simulink model "MPPT2"  (R2018b)
settings: Solver=ode23tb  StartTime=0.0  StopTime=inf  MaxStep=1e-4  RelTol=1e-3
PreLoadFcn:
  | load('EmulatedPV_LowPowerData.mat');
  | 
  | numIrr = 10;
  | ArrayPower = ArrayCurrent.*ArrayVoltage;
InitFcn:
  | Ts = 1e-4;
  | Tc = Ts;
undefined symbols (not defined in the file): ArrayCurrent, ArrayVoltage, DiscIntNeverNeededParam, Irradiance
libraries: powerlib x11
settings Model: Creator=mmishra  LastModifiedBy=malshikhkhalil
settings DebuggingCC: LibraryContextMissingDiagnostic=none
settings SFSimCC: SimUseLocalCustomCode=off
settings RTWCC: RTWUseLocalCustomCode=off

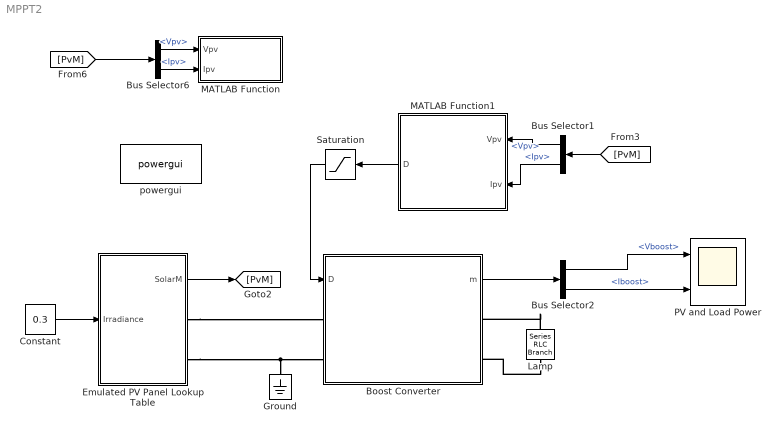
== system MPPT2 ==
  Boost Converter : Subsystem
  Bus Selector1 : BusSelector  OutputSignals=Vpv,Ipv
  Bus Selector2 : BusSelector  OutputSignals=Vboost,Iboost
  Bus Selector6 : BusSelector  OutputSignals=Vpv,Ipv
  Constant : Constant  Value=0.3
  Emulated PV Panel Lookup Table : Subsystem
      mask Display:
      | image(imread('panel.jpg'))
      | color('yellow')
      | port_label('input',1,'Ir')
      | port_label('output',1,'m')
      | port_label('Rconn',1,'A')
      | port_label('Rconn',2,'B')
  Ground : powerlib/Elements/Ground  LConnTagsString=a
      settings: SourceProductName=Simscape Electrical
  Lamp : powerlib/Elements/Series RLC Branch  LConnTagsString=__new0  RConnTagsString=__new0  BranchType=R  Resistance=11.5  Inductance=1e-3  SetiL0=off  InitialCurrent=0  Capacitance=1e-6  Setx0=off  InitialVoltage=0  Measurements=None
      settings: SourceProductName=Simscape Electrical
  MATLAB Function : MATLAB Function  TreatAsAtomicUnit=on  SystemSampleTime=1/20
  MATLAB Function1 : MATLAB Function  TreatAsAtomicUnit=on
  PV and Load Power : Scope  NumInputPorts=2
  Saturation : Saturate  UpperLimit=1  LowerLimit=0
  powergui : powerlib/powergui  Priority=1  SimulationMode=Discrete  SampleTime=Ts  frequency=60  Iterations=50  frequencyindice=0  Pbase=100e6  ErrMax=1e-4  UnitsV=kV  UnitsW=MW  buscounter=0  FunctionMessages=off  echomessages=off  EnableUseOfTLC=off  CurrentSourceSwitches=off  DisableSnubberDevices=off  DisableRonSwitches=off  DisableVfSwitches=off  DisplayEquations=off  SolverType=Tustin/Backward Euler (TBE)  Interpol=off  ExternalGateDelay=off  methode=off  Ts=100  x0status=blocks  SPID=on  SwTol=0  HookPort=off  RestoreLinks=warning  ResistiveCurrentMeasurement=off  Frange=[0:2:500]  Ylog=off  Xlog=on  ShowGrid=off  save=off  variable=ZData  structure=0  ZoomFFT=off  StartTime=0.0  cycles=1  DisplayStyle=1  fundamental=60  FreqAxis=off  MaxFrequency=1000  frequencyindicesteady=1  RmsSteady=1  display=off
  wires:
  Constant/1 -> Emulated PV Panel Lookup Table/1(Irradiance)
  Emulated PV Panel Lookup Table/1(SolarM) -> [PvM]
  Boost Converter/1(m) -> Bus Selector2/1
  Bus Selector6/1 -> MATLAB Function/1(Vpv)  "<Vpv>"
  Bus Selector6/2 -> MATLAB Function/2(Ipv)  "<Ipv>"
  [PvM] -> Bus Selector6/1
  MATLAB Function1/1(D) -> Saturation/1
  Saturation/1 -> Boost Converter/1(D)
  [PvM] -> Bus Selector1/1
  Bus Selector1/1 -> MATLAB Function1/1(Vpv)  "<Vpv>"
  Bus Selector1/2 -> MATLAB Function1/2(Ipv)  "<Ipv>"
  Bus Selector2/1 -> PV and Load Power/1  "<Vboost>"
  Bus Selector2/2 -> PV and Load Power/2  "<Iboost>"
  connections:
  Ground/LConn1 -- Emulated PV Panel Lookup Table/RConn2 -- Boost Converter/LConn2
  Emulated PV Panel Lookup Table/RConn1 -- Boost Converter/LConn1
  Lamp/LConn1 -- Boost Converter/RConn1
  Lamp/RConn1 -- Boost Converter/RConn2

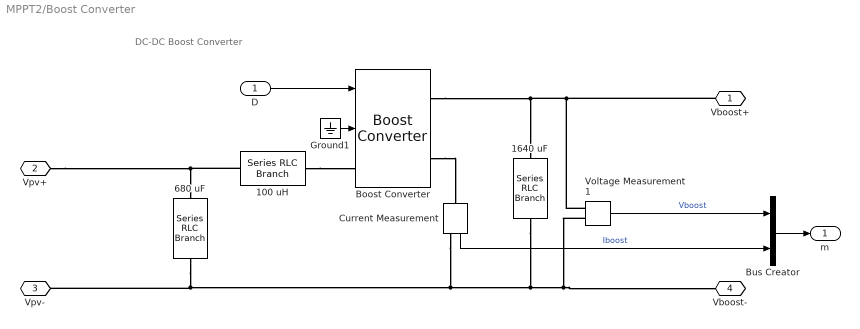
== system MPPT2/Boost Converter ==
  note: DC-DC Boost Converter
  D : Inport
  100 uH : powerlib/Elements/Series RLC Branch  LConnTagsString=__new0  RConnTagsString=__new0  BranchType=L  Resistance=1  Inductance=100e-6  SetiL0=off  InitialCurrent=0  Capacitance=1e-6  Setx0=off  InitialVoltage=0  Measurements=None
      settings: SourceProductName=Simscape Electrical
  1640 uF : powerlib/Elements/Series RLC Branch  LConnTagsString=__new0  RConnTagsString=__new0  BranchType=C  Resistance=1  Inductance=1e-3  SetiL0=off  InitialCurrent=0  Capacitance=1640e-6  Setx0=off  InitialVoltage=30  Measurements=None
      settings: SourceProductName=Simscape Electrical
  680 uF : powerlib/Elements/Series RLC Branch  LConnTagsString=__new0  RConnTagsString=__new0  BranchType=C  Resistance=1e-3  Inductance=1e-3  SetiL0=off  InitialCurrent=0  Capacitance=680e-6  Setx0=off  InitialVoltage=20  Measurements=None
      settings: SourceProductName=Simscape Electrical
  "Boost Converter " : powerlib/Power Electronics/Boost Converter  ModelType=Average model (D-controlled)  Ron=1e-3  Rs=1e6  Cs=inf  Vforward=[0,0.8]  Ron_Diode=1e-3  Rs_Diode=1e6  Cs_Diode=inf  Vf_Diode=0.8  Rs_CurrentSource=inf
      settings: SourceProductName=Simscape Electrical  SourceProductBaseCode=PS
  Bus Creator : BusCreator  Inputs=2
  Current Measurement : powerlib/Measurements/Current Measurement  PhasorSimulation=off  OutputType=Complex  PSBequivalent=0
      settings: SourceProductName=Simscape Electrical
  Ground1 : Ground
  Voltage Measurement1 : powerlib/Measurements/Voltage Measurement  PhasorSimulation=off  OutputType=Complex  PSBequivalent=0
      settings: SourceProductName=Simscape Electrical
  Vboost+ : PMIOPort  Side=Right
  Vpv+ : PMIOPort  Port=2  Side=Left
  Vpv- : PMIOPort  Port=3  Side=Left
  Vboost- : PMIOPort  Port=4  Side=Right
  m : Outport
  wires:
  Ground1/1 -> "Boost Converter "/2
  Bus Creator/1 -> m/1
  Voltage Measurement1/1 -> Bus Creator/1  "Vboost"
  Current Measurement/1 -> Bus Creator/2  "Iboost"
  D/1 -> "Boost Converter "/1
  connections:
  100 uH/LConn1 -- Vpv+/RConn1 -- 680 uF/LConn1
  "Boost Converter "/RConn2 -- Current Measurement/LConn1
  100 uH/RConn1 -- "Boost Converter "/LConn1
  Voltage Measurement1/LConn1 -- Vboost+/RConn1 -- "Boost Converter "/RConn1 -- 1640 uF/LConn1
  680 uF/RConn1 -- Vboost-/RConn1 -- Voltage Measurement1/LConn2 -- 1640 uF/RConn1 -- Current Measurement/RConn1 -- Vpv-/RConn1

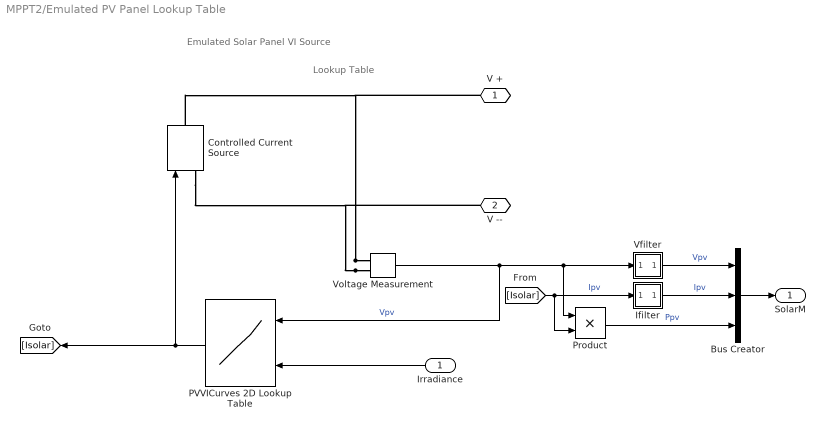
== system MPPT2/Emulated PV Panel Lookup Table ==
  note: Lookup Table
  note: Emulated Solar Panel VI Source
  Irradiance : Inport
  Bus Creator : BusCreator  Inputs=3
  Controlled Current Source : powerlib/Electrical Sources/Controlled Current Source  Initialize=on  Source_Type=AC  Amplitude=0  Phase=0  Frequency=0  Measurements=None
      settings: SourceProductName=Simscape Electrical
  Ifilter : Subsystem  mask{Tf=0.01}
      mask prompts: Tf "Filter Time Constant"
  PVVICurves 2D Lookup Table : Lookup_n-D  BreakpointsForDimension1=ArrayVoltage  BreakpointsForDimension2=Irradiance  Table=ArrayCurrent  InternalRulePriority=Speed  RndMeth=Simplest  InputSameDT=on
  Product : Product
  Vfilter : Subsystem  mask{Tf=0.01}
      mask prompts: Tf "Filter Time Constant"
  Voltage Measurement : powerlib/Measurements/Voltage Measurement  PhasorSimulation=off  OutputType=Complex  PSBequivalent=0
      settings: SourceProductName=Simscape Electrical
  V + : PMIOPort  Side=Right
  V -- : PMIOPort  Port=2  Side=Right
  SolarM : Outport
  wires:
  Irradiance/1 -> PVVICurves 2D Lookup Table/2
  Bus Creator/1 -> SolarM/1
  [Isolar] -> Product/2, Ifilter/1(u)  "Ipv"
  Product/1 -> Bus Creator/3  "Ppv"
  PVVICurves 2D Lookup Table/1 -> [Isolar], Controlled Current Source/1
  Voltage Measurement/1 -> Product/1, Vfilter/1(u), PVVICurves 2D Lookup Table/1  "Vpv"
  Vfilter/1(y) -> Bus Creator/1  "Vpv"
  Ifilter/1(y) -> Bus Creator/2  "Ipv"
  connections:
  Voltage Measurement/LConn2 -- Controlled Current Source/LConn1 -- V --/RConn1
  Voltage Measurement/LConn1 -- Controlled Current Source/RConn1 -- V +/RConn1

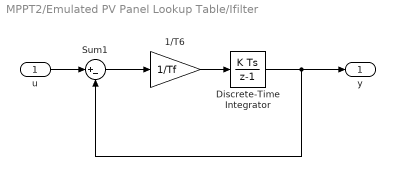
== system MPPT2/Emulated PV Panel Lookup Table/Ifilter ==
  u : Inport
  1/T6 : Gain  Gain=1/Tf
  Discrete-Time Integrator : DiscreteIntegrator  SampleTime=Tc  ICPrevOutput=DiscIntNeverNeededParam  ICPrevScaledInput=DiscIntNeverNeededParam
  Sum1 : Sum  Inputs=|+-
  y : Outport
  wires:
  Sum1/1 -> 1/T6/1
  Discrete-Time Integrator/1 -> Sum1/2, y/1
  u/1 -> Sum1/1
  1/T6/1 -> Discrete-Time Integrator/1

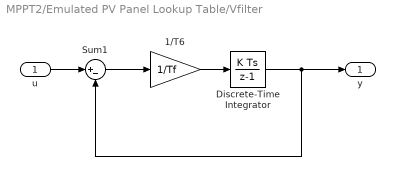
== system MPPT2/Emulated PV Panel Lookup Table/Vfilter ==
  u : Inport
  1/T6 : Gain  Gain=1/Tf
  Discrete-Time Integrator : DiscreteIntegrator  SampleTime=Tc  ICPrevOutput=DiscIntNeverNeededParam  ICPrevScaledInput=DiscIntNeverNeededParam
  Sum1 : Sum  Inputs=|+-
  y : Outport
  wires:
  1/T6/1 -> Discrete-Time Integrator/1
  u/1 -> Sum1/1
  Discrete-Time Integrator/1 -> y/1, Sum1/2
  Sum1/1 -> 1/T6/1

== matlab function MPPT2/MATLAB Function1 ==
  data: Vpv input; D output; Ipv input
function D=Pando(Vpv,Ipv)
%Perturb and Observe algorithm
% for Maximum Power Point Tracking.

% Define internal values for voltage and power as persistent 
% variables
persistent Dprev Pprev Vprev

%Initialize the internal values for the voltage and power on the
% first pass
if isempty(Dprev)
    Dprev = 0.7;
    Vprev = 190;
    Pprev = 2000;
end

% Initialize algorithm parameters
deltaD = 0.001;

% Calculate measured array power
Ppv = Vpv*Ipv;

%Increase or decrease duty cycle based on conditions
if (Ppv-Pprev) ~=0
    if (Ppv-Pprev) > 0
        if (Vpv-Vprev) >0
            D = Dprev-deltaD;
        else
            D = Dprev+deltaD;
        end
    else
        if (Vpv-Vprev)>0
            D=Dprev+deltaD;
        else
            D = Dprev-deltaD;
        end
    end
else
    D=Dprev;
end
% Update internal values
Dprev =D;
Vprev =Vpv;
Pprev = Ppv;

== matlab function MPPT2/MATLAB Function ==
  settings: updateMethod=DISCRETE
  data: Vpv input; Ipv input; ArrayPower parameter; ArrayVoltage parameter; numIrr parameter
function plotPower(Vpv,Ipv, ArrayPower,ArrayVoltage, numIrr)

    persistent irrPlot powerPlot
%     coder.extrinsic('legend');    
    
    if isempty(irrPlot)
        
        idx = 1:find(ArrayPower(:,numIrr) > 0,1,'last')+2;
                        
        figure(1);
        irrPlot = plot(ArrayVoltage(idx),ArrayPower(idx,1:numIrr)); hold on;
        grid on;
        
        xlabel('PV Voltage [V]');
        ylabel('PV Power [W]');
        title('PV Power Output');
        
        powerPlot = plot(Vpv,Vpv*Ipv,'ro'); 
%         legend('50 W/m^2','100 W/m^2','150 W/m^2','200 W/m^2','250 W/m^2','300 W/m^2',...
%             '350 W/m^2','400 W/m^2','450 W/m^2','500 W/m^2','PV Power');
        hold off;
        
    else 
        set(powerPlot,'XData',Vpv,'YData',Vpv*Ipv);
    end
    
end
